simulink model "sampleModel"  (R2021a)
settings: Solver=VariableStepAuto  StartTime=0.0  StopTime=10.0  RelTol=1e-3
settings Model: Creator=ECHOLODO  LastModifiedBy=20204920
settings SolverCC: AlgebraicLoopSolver=TrustRegion
settings DebuggingCC: SFMachineParentedDataDiag=warning

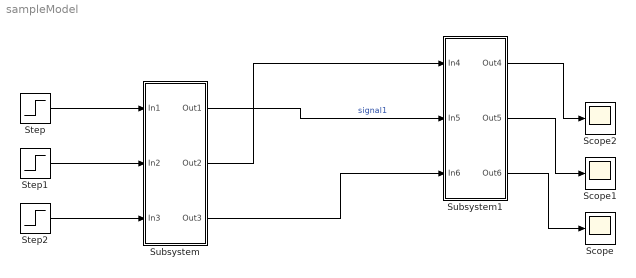
== system sampleModel ==
  Scope : Scope
  Scope1 : Scope
  Scope2 : Scope
  Step : Step  SampleTime=0
  Step1 : Step  SampleTime=0
  Step2 : Step  SampleTime=0
  Subsystem : Subsystem
  Subsystem1 : Subsystem
  wires:
  Step/1 -> Subsystem/1(In1)
  Step1/1 -> Subsystem/2(In2)
  Step2/1 -> Subsystem/3(In3)
  Subsystem1/2(Out5) -> Scope1/1
  Subsystem1/3(Out6) -> Scope/1
  Subsystem1/1(Out4) -> Scope2/1
  Subsystem/1(Out1) -> Subsystem1/2(In5)  "signal1"
  Subsystem/3(Out3) -> Subsystem1/3(In6)
  Subsystem/2(Out2) -> Subsystem1/1(In4)

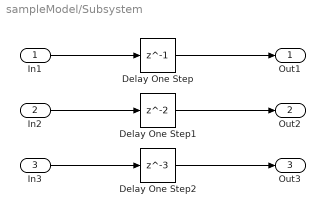
== system sampleModel/Subsystem ==
  In1 : Inport
  In2 : Inport  Port=2
  In3 : Inport  Port=3
  Delay One Step : Delay  DelayLength=1
  Delay One Step1 : Delay
  Delay One Step2 : Delay  DelayLength=3
  Out1 : Outport
  Out2 : Outport  Port=2
  Out3 : Outport  Port=3
  wires:
  Delay One Step/1 -> Out1/1
  In1/1 -> Delay One Step/1
  In3/1 -> Delay One Step2/1
  Delay One Step1/1 -> Out2/1
  In2/1 -> Delay One Step1/1
  Delay One Step2/1 -> Out3/1

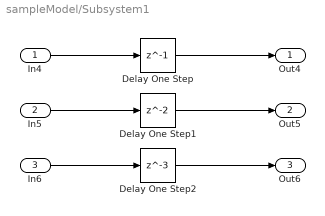
== system sampleModel/Subsystem1 ==
  In4 : Inport
  In5 : Inport  Port=2
  In6 : Inport  Port=3
  Delay One Step : Delay  DelayLength=1
  Delay One Step1 : Delay
  Delay One Step2 : Delay  DelayLength=3
  Out4 : Outport
  Out5 : Outport  Port=2
  Out6 : Outport  Port=3
  wires:
  Delay One Step/1 -> Out4/1
  In4/1 -> Delay One Step/1
  In6/1 -> Delay One Step2/1
  Delay One Step1/1 -> Out5/1
  In5/1 -> Delay One Step1/1
  Delay One Step2/1 -> Out6/1
